simulink model "analysis_discrete_hinf_ctrl_lin_uncertain_model_z"  (R2020b)
settings: Solver=VariableStepAuto  StartTime=0.0  StopTime=10.0  RelTol=1e-3
values from neighbouring files (symbols this model uses):
  B = 10    [hinfCostFunc.m]    (also in hinf_analysis_z.m = 11; hinf_cmd_lmi.m = [zeros(4,2); Sigma.B]; init_rob_synth_sim.m; muCostFunc.m = 11)
  dq0 = [0;0;0]    [hinfCostFunc.m]    (also in hinf_analysis_z.m; init_rob_synth_sim.m = [0; 0; 0]; muCostFunc.m; mu_analysis_z.m)
  M = 0.45    [hinfCostFunc.m]    (also in hinf_analysis_z.m = 0.42; init_rob_synth_sim.m; muCostFunc.m = 0.42; mu_analysis_z.m = 0.42)
  q0 = [1.676; -4.363; 1.497]    [hinfCostFunc.m]    (also in hinf_analysis_z.m; init_rob_synth_sim.m; muCostFunc.m; mu_analysis_z.m)
  Sigma = minreal(Sigma, [], false)    [hinfCostFunc.m]    (also in hinf_analysis_z.m = youbot_lin_model_ss_z; hinf_cmd_lmi.m = youbot_lin_model_ss_z; muCostFunc.m; mu_analysis_z.m = youbot_lin_model_ss_z)
  tau_m = 1/(10*2*pi)    (= 0.0159154943092)    [hinfCostFunc.m]    (also in hinf_analysis_z.m; init_rob_synth_sim.m; muCostFunc.m; mu_analysis_z.m)
libraries: cstblocks x1, RCTblocks x1
settings Model: Creator=fortineau_vin  LastModifiedBy=fortineau_vin

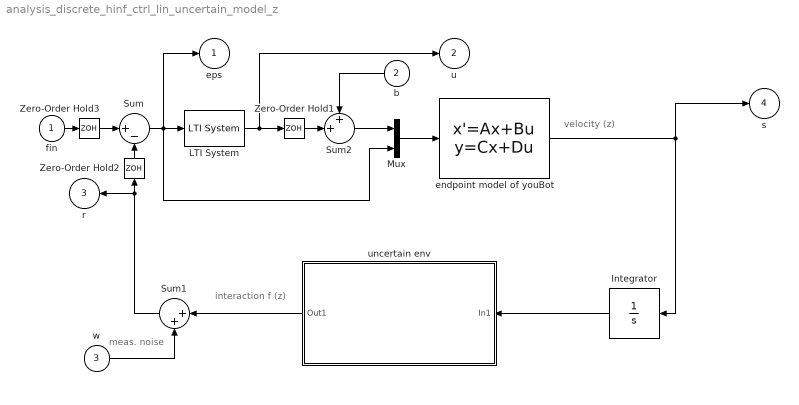
== system analysis_discrete_hinf_ctrl_lin_uncertain_model_z ==
  note: meas. noise
  note: interaction f (z)
  note: velocity (z)
  fin : Inport  PortDimensions=1
  b : Inport  Port=2  PortDimensions=1
  w : Inport  Port=3  PortDimensions=1
  Integrator : Integrator
  LTI System : cstblocks/LTI System  sys=Hinf_ctrl_red_dis  IC=[]
  Mux : Mux  Inputs=2
  Sum : Sum  Inputs=|+-
  Sum1 : Sum  Inputs=|++
  Sum2 : Sum  Inputs=++|
  Zero-Order Hold1 : ZeroOrderHold  SampleTime=-1
  Zero-Order Hold2 : ZeroOrderHold  SampleTime=-1
  Zero-Order Hold3 : ZeroOrderHold  SampleTime=-1
  endpoint model of youBot : StateSpace  A=Sigma.A  B=Sigma.B  C=Sigma.C  D=Sigma.D  InitialCondition=[q0;dq0]
  uncertain env : Subsystem
  eps : Outport  PortDimensions=1
  u : Outport  Port=2  PortDimensions=1
  r : Outport  Port=3  PortDimensions=1
  s : Outport  Port=4  PortDimensions=1
  wires:
  Zero-Order Hold2/1 -> Sum/2
  fin/1 -> Zero-Order Hold3/1
  w/1 -> Sum1/2
  Sum1/1 -> Zero-Order Hold2/1, r/1
  b/1 -> Sum2/1
  Mux/1 -> endpoint model of youBot/1
  LTI System/1 -> Zero-Order Hold1/1, u/1
  Zero-Order Hold1/1 -> Sum2/2
  Sum2/1 -> Mux/1
  Sum/1 -> LTI System/1, eps/1, Mux/2
  Zero-Order Hold3/1 -> Sum/1
  endpoint model of youBot/1 -> s/1, Integrator/1
  Integrator/1 -> uncertain env/1(In1)
  uncertain env/1(Out1) -> Sum1/1

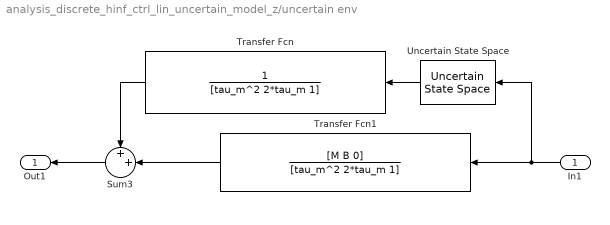
== system analysis_discrete_hinf_ctrl_lin_uncertain_model_z/uncertain env ==
  In1 : Inport
  Sum3 : Sum  Inputs=++|
  Transfer Fcn : TransferFcn  Denominator=[tau_m^2 2*tau_m 1]
  Transfer Fcn1 : TransferFcn  Numerator=[M B 0]  Denominator=[tau_m^2 2*tau_m 1]
  Uncertain State Space : RCTblocks/Uncertain State Space  Tag=USS  USystem=K  UValue=[]  X0=[]  uX0=[]
      settings: SourceProductBaseCode=RC
  Out1 : Outport
  wires:
  Transfer Fcn/1 -> Sum3/1
  Sum3/1 -> Out1/1
  In1/1 -> Transfer Fcn1/1, Uncertain State Space/1
  Transfer Fcn1/1 -> Sum3/2
  Uncertain State Space/1 -> Transfer Fcn/1
